simulink model "ThdRwLtStBkReclnHolderChk"  (R2018b)
settings: Solver=FixedStepDiscrete  StartTime=0.0  StopTime=10.0  FixedStep=0.01  RelTol=1e-3
libraries: simulink x1
settings Model: Creator=sn2xws  LastModifiedBy=sn2xws
settings DataIOCC: SaveFormat=StructureWithTime
settings OptimizationCC: DefaultParameterBehavior=Inlined  EnhancedBackFolding=on  PassReuseOutputArgsAs=Individual arguments  ZeroExternalMemoryAtStartup=off  ZeroInternalMemoryAtStartup=off  OptimizeBlockOrder=speed  DifferentSizesBufferReuse=on  OptimizationCustomize=off
settings DebuggingCC: ParameterTunabilityLossMsg=error
settings ModelReferenceCC: ModelReferenceNumInstancesAllowed=Single
settings SFSimCC: MATLABDynamicMemAlloc=off
settings RTWCC: SystemTargetFile=autosar.tlc  GenCodeOnly=on  TemplateMakefile=ert_default_tmf  Description=AUTOSAR  GenerateReport=on  IncludeHyperlinkInReport=on  LaunchReport=on  GenerateTraceInfo=on  GenerateTraceReport=on  GenerateTraceReportSl=on  GenerateTraceReportSf=on  GenerateTraceReportEml=on
settings CodeAppCC: ForceParamTrailComments=on  IgnoreCustomStorageClasses=off  OperatorAnnotations=on  SimulinkDataObjDesc=on  SFDataObjDesc=on  InsertBlockDesc=on
settings STFCustomTargetCC: TargetLangStandard=C99 (ISO)  MultiwordLength=256  ParMdlRefBuildCompliant=on  CompOptLevelCompliant=on  IncludeMdlTerminateFcn=off  CombineOutputUpdateFcns=on  SuppressErrorStatus=on  ERTCustomFileBanners=on  SupportNonFinite=off  SupportComplex=off  SupportContinuousTime=off  SupportNonInlinedSFcns=off  RemoveResetFunc=on  MATLABClassNameForMDSCustomization=Simulink.SoftwareTarget.ERTCustomization  AutosarCompliant=on  UseToolchainInfoCompliant=on  LookupTableObjectStructAxisOrder=2,1,3,4,...  LUTObjectStructOrderEvenSpacing=Size,Table,Breakpoints  SystemTargetFile=autosar.tlc
settings ERTTargetCC: TargetLangStandard=C99 (ISO)  ConcurrentExecutionCompliant=off  IncludeMdlTerminateFcn=off  SuppressErrorStatus=on  SupportNonFinite=off  SupportComplex=off  ModelStepFunctionPrototypeControlCompliant=off  CPPClassGenCompliant=off  AutosarCompliant=on  LookupTableObjectStructAxisOrder=2,1,3,4,...  LUTObjectStructOrderEvenSpacing=Size,Table,Breakpoints  InlinedParameterPlacement=NonHierarchical  ERTCustomFileTemplate=example_file_process.tlc  ERTFilePackagingFormat=Compact

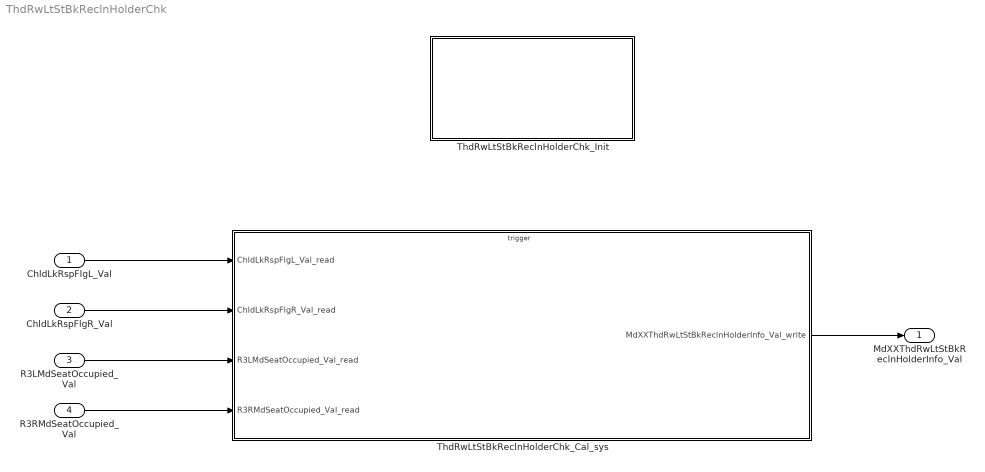
== system ThdRwLtStBkReclnHolderChk ==
  ChldLkRspFlgL_Val : Inport  OutDataTypeStr=boolean  PortDimensions=1
  ChldLkRspFlgR_Val : Inport  Port=2  OutDataTypeStr=boolean  PortDimensions=1
  R3LMdSeatOccupied_Val : Inport  Port=3  OutDataTypeStr=boolean  PortDimensions=1
  R3RMdSeatOccupied_Val : Inport  Port=4  OutDataTypeStr=boolean  PortDimensions=1
  ThdRwLtStBkReclnHolderChk_Cal_sys : Subsystem
  ThdRwLtStBkReclnHolderChk_Init : Subsystem
  MdXXThdRwLtStBkReclnHolderInfo_Val : Outport  OutDataTypeStr=uint32  PortDimensions=1
  wires:
  ChldLkRspFlgL_Val/1 -> ThdRwLtStBkReclnHolderChk_Cal_sys/1(ChldLkRspFlgL_Val_read)
  ChldLkRspFlgR_Val/1 -> ThdRwLtStBkReclnHolderChk_Cal_sys/2(ChldLkRspFlgR_Val_read)
  R3LMdSeatOccupied_Val/1 -> ThdRwLtStBkReclnHolderChk_Cal_sys/3(R3LMdSeatOccupied_Val_read)
  R3RMdSeatOccupied_Val/1 -> ThdRwLtStBkReclnHolderChk_Cal_sys/4(R3RMdSeatOccupied_Val_read)
  ThdRwLtStBkReclnHolderChk_Cal_sys/1(MdXXThdRwLtStBkReclnHolderInfo_Val_write) -> MdXXThdRwLtStBkReclnHolderInfo_Val/1

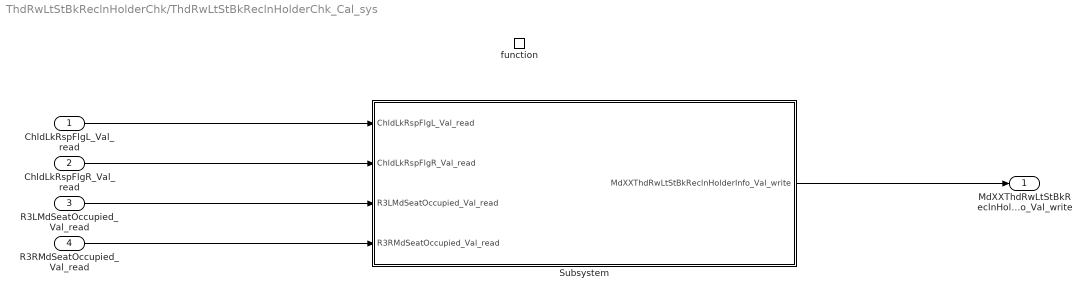
== system ThdRwLtStBkReclnHolderChk/ThdRwLtStBkReclnHolderChk_Cal_sys ==
  ChldLkRspFlgL_Val_read : Inport
  ChldLkRspFlgR_Val_read : Inport  Port=2
  R3LMdSeatOccupied_Val_read : Inport  Port=3
  R3RMdSeatOccupied_Val_read : Inport  Port=4
  function : TriggerPort  TriggerType=function-call  IsSimulinkFunction=on  FunctionName=ThdRwLtStBkReclnHolderChk_Cal  VariantControl=(inherit)
  Subsystem : Subsystem
  MdXXThdRwLtStBkReclnHolderInfo_Val_write : Outport
      settings: EnsureOutportIsVirtual=on
  wires:
  Subsystem/1(MdXXThdRwLtStBkReclnHolderInfo_Val_write) -> MdXXThdRwLtStBkReclnHolderInfo_Val_write/1
  ChldLkRspFlgL_Val_read/1 -> Subsystem/1(ChldLkRspFlgL_Val_read)
  ChldLkRspFlgR_Val_read/1 -> Subsystem/2(ChldLkRspFlgR_Val_read)
  R3LMdSeatOccupied_Val_read/1 -> Subsystem/3(R3LMdSeatOccupied_Val_read)
  R3RMdSeatOccupied_Val_read/1 -> Subsystem/4(R3RMdSeatOccupied_Val_read)

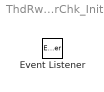
== system ThdRwLtStBkReclnHolderChk/ThdRwLtStBkReclnHolderChk_Init ==
  Event Listener : EventListener  EventName=reset

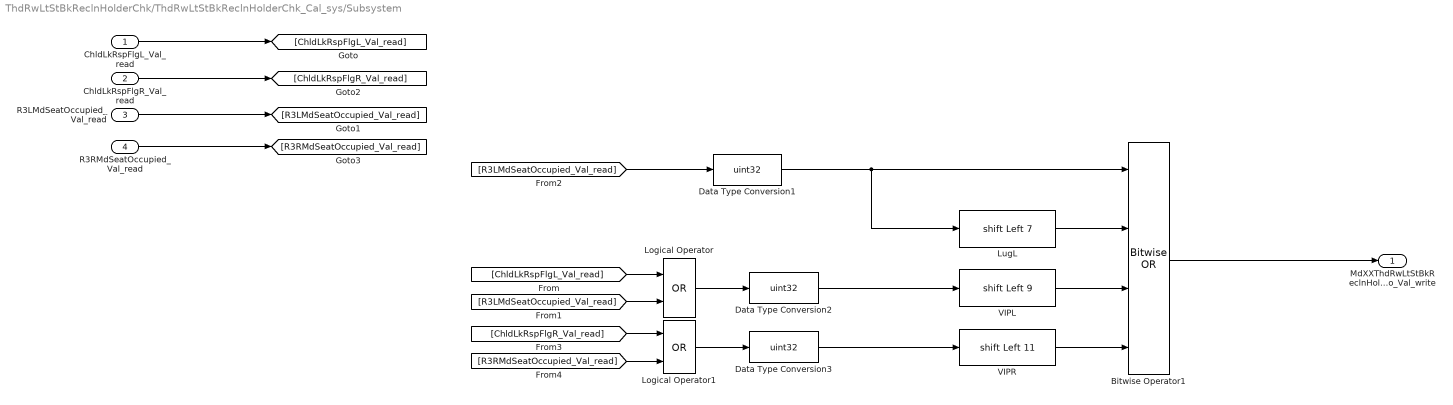
== system ThdRwLtStBkReclnHolderChk/ThdRwLtStBkReclnHolderChk_Cal_sys/Subsystem ==
  ChldLkRspFlgL_Val_read : Inport
  ChldLkRspFlgR_Val_read : Inport  Port=2
  R3LMdSeatOccupied_Val_read : Inport  Port=3
  R3RMdSeatOccupied_Val_read : Inport  Port=4
  Bitwise Operator1 : simulink/Logic and Bit Operations/Bitwise Operator  logicop=OR  UseBitMask=off  NumInputPorts=4  BitMask=bin2dec('11011001')  BitMaskRealWorld=Stored Integer
  Data Type Conversion1 : DataTypeConversion  OutDataTypeStr=uint32
  Data Type Conversion2 : DataTypeConversion  OutDataTypeStr=uint32
  Data Type Conversion3 : DataTypeConversion  OutDataTypeStr=uint32
  Logical Operator : Logic  Operator=OR  AllPortsSameDT=off  OutDataTypeStr=boolean
  Logical Operator1 : Logic  Operator=OR  AllPortsSameDT=off  OutDataTypeStr=boolean
  LugL : ArithShift  BitShiftNumber=7  BitShiftDirection=Left
  VIPL : ArithShift  BitShiftNumber=9  BitShiftDirection=Left
  VIPR : ArithShift  BitShiftNumber=11  BitShiftDirection=Left
  MdXXThdRwLtStBkReclnHolderInfo_Val_write : Outport
      settings: EnsureOutportIsVirtual=on
  wires:
  Bitwise Operator1/1 -> MdXXThdRwLtStBkReclnHolderInfo_Val_write/1
  R3RMdSeatOccupied_Val_read/1 -> [R3RMdSeatOccupied_Val_read]
  ChldLkRspFlgR_Val_read/1 -> [ChldLkRspFlgR_Val_read]
  ChldLkRspFlgL_Val_read/1 -> [ChldLkRspFlgL_Val_read]
  R3LMdSeatOccupied_Val_read/1 -> [R3LMdSeatOccupied_Val_read]
  [R3LMdSeatOccupied_Val_read] -> Data Type Conversion1/1
  Data Type Conversion1/1 -> LugL/1, Bitwise Operator1/1
  LugL/1 -> Bitwise Operator1/2
  [ChldLkRspFlgL_Val_read] -> Logical Operator/1
  [R3LMdSeatOccupied_Val_read] -> Logical Operator/2
  Logical Operator/1 -> Data Type Conversion2/1
  Data Type Conversion2/1 -> VIPL/1
  VIPL/1 -> Bitwise Operator1/3
  [ChldLkRspFlgR_Val_read] -> Logical Operator1/1
  [R3RMdSeatOccupied_Val_read] -> Logical Operator1/2
  Logical Operator1/1 -> Data Type Conversion3/1
  Data Type Conversion3/1 -> VIPR/1
  VIPR/1 -> Bitwise Operator1/4
